simulink model "ej5_2"  (R2023a)
settings: Solver=VariableStepAuto  StartTime=0.0  StopTime=4  MaxStep=1e-4  RelTol=1e-3
libraries: SignalEditorBlockLib x2
settings Model: Creator=Juan  LastModifiedBy=Juan

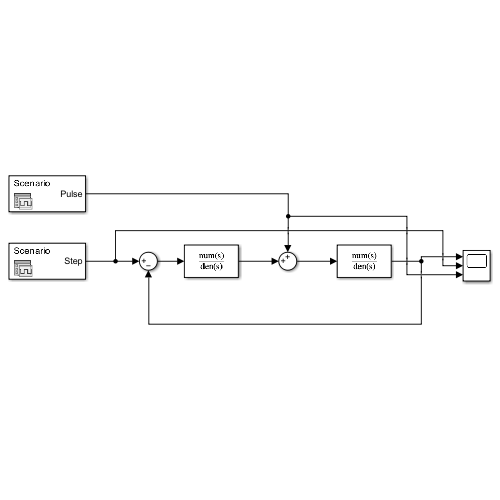
[thumbnail: Simulink's stored preview of the top-level diagram]
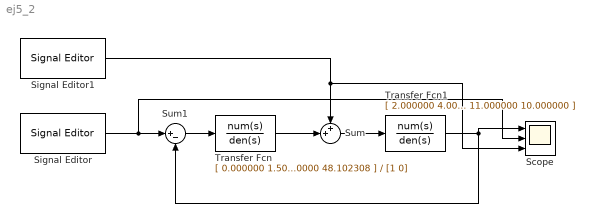
== system ej5_2 ==
  Scope : Scope  NumInputPorts=3
  Signal Editor : SignalEditorBlockLib/Signal Editor  FileName=D:\01. Facultad\Control y Sistemas1\Control y Sistemas\Tp8\ref.mat  ActiveScenario=Scenario  ActiveSignal=Step  IsBus=off  OutputBusObjectStr=Bus: BusObject  SampleTime=0  Interpolate=off  ZeroCross=off  OutputAfterFinalValue=Setting to zero  Unit=inherit  PreserveSignalName=on  ApplySigPropsToAllScenarios=on
  Signal Editor1 : SignalEditorBlockLib/Signal Editor  FileName=D:\01. Facultad\Control y Sistemas1\Control y Sistemas\Tp8\untitled.mat  ActiveScenario=Scenario  ActiveSignal=Pulse  IsBus=off  OutputBusObjectStr=Bus: BusObject  SampleTime=0  Interpolate=off  ZeroCross=off  OutputAfterFinalValue=Setting to zero  Unit=inherit  PreserveSignalName=on  ApplySigPropsToAllScenarios=on
  Sum : Sum  Inputs=++|
  Sum1 : Sum  Inputs=|+-
  Transfer Fcn : TransferFcn  Numerator=[ 0.000000 1.500000 48.102308 ]  Denominator=[1 0]
  Transfer Fcn1 : TransferFcn  Numerator=[ 2.000000 4.000000 ]  Denominator=[ 1.000000 11.000000 10.000000 ]
  wires:
  Signal Editor1/1 -> Scope/3, Sum/1
  Transfer Fcn/1 -> Sum/2
  Sum/1 -> Transfer Fcn1/1
  Transfer Fcn1/1 -> Scope/1, Sum1/2
  Signal Editor/1 -> Scope/2, Sum1/1
  Sum1/1 -> Transfer Fcn/1
